simulink model "compare"  (R2025b)
settings: Solver=ode23t  StartTime=0.0  StopTime=4  RelTol=1e-2  AbsTol=1e-2  EnableMultiTasking=on
values from neighbouring files (symbols this model uses):
  k = 2    [compare_init.m]
  N = numel(knee_data)    [display_imu_measurements.m]
  time = 0.08    [compare_init.m]
  X = zeros(N,1)    [display_imu_measurements.m]
  Z = zeros(N,1)    [display_imu_measurements.m]
undefined symbols (not defined in the file or in its folder): foot_radius, ground_offset, hip_max_angle, hip_min_angle, Kaction, knee_max_angle, knee_min_angle, Kpitch, Kroll, Kt, Kv1, Kv2, Ky, Kz, lower_leg, max_a, max_friction_force, max_hip_speed, max_knee_speed, max_magnitude_force, max_torque, max_v, point1, point2, point3, point4, robot_offset, T, Tf, torso, upper_leg, Y
libraries: nesl_utility x88, sm_lib x66, rllib x1
(part 1 of 4)
settings Model: Creator=filip  LastModifiedBy=filip
settings SolverCC: ZeroCrossAlgorithm=Adaptive  MaxZcPerStep=1.0
settings DataIOCC: LimitDataPoints=on  MaxDataPoints=10000
settings OptimizationCC: ReuseModelBlockBuffer=off  LifeSpan=inf
settings DebuggingCC: AlgebraicLoopMsg=none  UnconnectedInputMsg=warning  UnconnectedOutputMsg=warning  UnconnectedLineMsg=warning  AllowSymbolicDim=off  SubsystemReferenceDiagnosticForUnitTest=warning  SFUnexpectedBacktrackingDiag=warning  SFNoUnconditionalDefaultTransitionDiag=warning  SFExecutionAtInitializationDiag=none  ArithmeticOperatorsInVariantConditions=warning
settings ModelReferenceCC: EnableRefExpFcnMdlSchedulingChecks=on
settings SFSimCC: SimUseLocalCustomCode=off  CustomCodeUndefinedFunction=UseInterfaceOnly
settings RTWCC: RTWUseLocalCustomCode=off  GPUComputeCapability=3.5  DLArmComputeVersion=19.05
settings CodeAppCC: StateflowObjectComments=on
settings GRTTargetCC: TargetLangStandard=C89/C90 (ANSI)
settings ConfigComp: CovMetricSettings=dw  CovSaveCumulativeToWorkspaceVar=on  CovSaveSingleToWorkspaceVar=on  CovExternalEMLEnable=off  CovSFcnEnable=off
settings SimscapeCC: SimscapeLogType=all  SimscapeLogSimulationStatistics=on  SimscapeLogDataHistory=10000.0
settings ExplorerConfigSet: InternalSimMechanicsExplorerSettings=|
  | <ExplorerConfiguration>
  | 
  |   <canonicalview>default</canonicalview>
  | 
  |   <TilePanel>
  |     <TileInfo>
  |       <Tiles Columns="1" Count="1" Height="896" Rows="1" Width="1591">
  |         <Row Weight="1"/>
  |         <Column Weight="1"/>
  |         <Tile Height="1" Width="1" X="0" Y="0"/>
  |       </Tiles>
  |     </TileInfo>
  |     <SceneInfo>
  |       <SceneViewer>
  |         <IsThisViewStd>
  |           <IsStandardView>off</IsStandardView>
  |           <StandardViewName>Front</StandardViewName>
  |         </IsThisViewStd>
  |         <BGColor>
  |           <R>1</R>
  |           <G>1</G>
  |           <B>1</B>
  |           <A>1</A>
  |         </BGColor>
  |         <Camera>
  |           <DoPerspective>off</DoPerspective>
  |           <Position>
  |             <X>2.3240540663599489</X>
  |             <Y>-79.864795009647452</Y>
  |             <Z>11.89876292667747</Z>
  |           </Position>
  |           <Center>
  |             <X>0.21287692287567161</X>
  |             <Y>-0.00025892895920284764</Y>
  |             <Z>-0.038859645903780687</Z>
  |           </Center>
  |           <Up>
  |             <X>-0.0013697347920566083</X>
  |             <Y>0.14779550973246389</Y>
  |             <Z>0.98901699233608753</Z>
  |           </Up>
  |           <XLim>0.21304392253015453</XLim>
  |           <YLim>0.21304392253015453</YLim>
  |           <ViewLimDist>0.01</ViewLimDist>
  |         </Camera>
  |       </SceneViewer>
  |     </SceneInfo>
  |   </TilePanel>
  | 
  |   <MechEditorPanel>
  |     <GfxPanelCameraMap/>
  |     <Cameras/>
  |     <VideoCreator>
  |       <IncludeTiles>All</IncludeTiles>
  |       <IncludeTime>on</IncludeTime>
  |       <IncludeWorldFrame>off</IncludeWorldFrame>
  |       <PlaybackSpeedRatio>1</PlaybackSpeedRatio>
  |       <FrameRate>30</FrameRate>
  |       <FrameSize>auto</FrameSize>
  |       <VideoFormat>UncompressedAVI</VideoFormat>
  |     </VideoCreator>
  |   </MechEditorPanel>
  | 
  |   <PlaybackSettings>
  |     <PlaybackSpeedFactor>1</PlaybackSpeedFactor>
  |   </PlaybackSettings>
  | 
  | </ExplorerConfiguration>

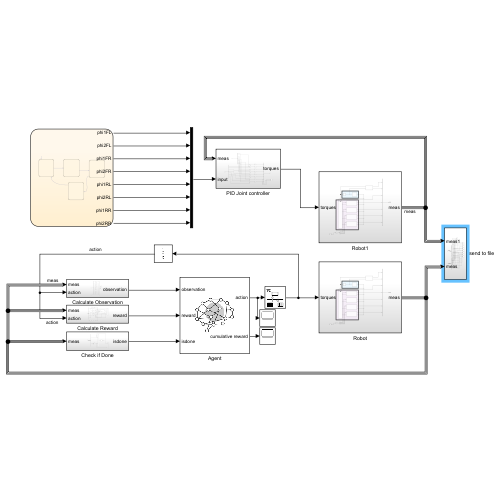
[thumbnail: Simulink's stored preview of the top-level diagram]
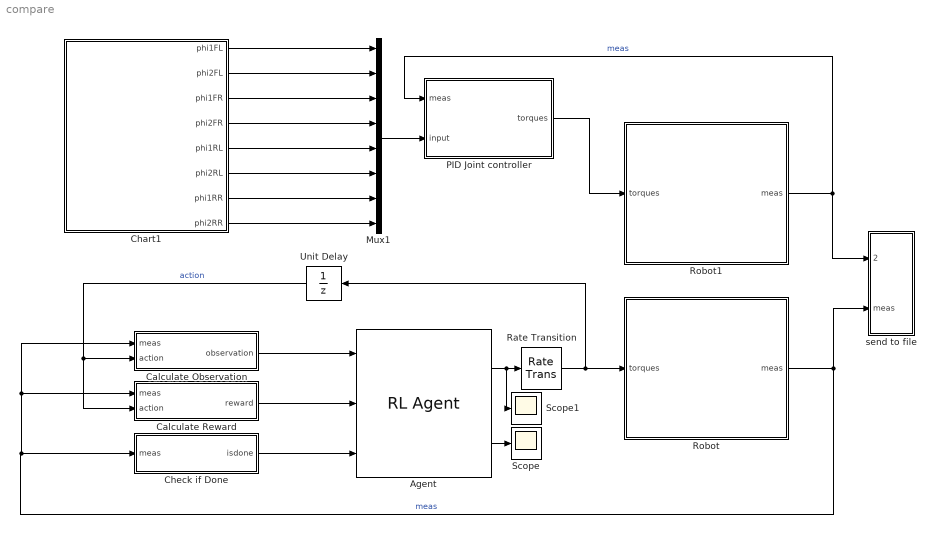
== system compare ==
  Agent : rllib/RL Agent  Agent=agent  ExternalActionAsInput=off  ProvideLastAction=off  ProvideCumRwd=on  TreatAsDirectFeedthrough=on  UseStrictObservationDataTypes=off
  Calculate Observation : Subsystem
  Calculate Reward : Subsystem
  Chart1 : Stateflow chart  TreatAsAtomicUnit=on
  Check if Done : Subsystem
  Mux1 : Mux  Inputs=8
  PID Joint controller : Subsystem
  Rate Transition : RateTransition
  Robot : Subsystem
  Robot1 : Subsystem
  Scope : Scope
      settings: ActiveDisplayYMinimum=-401.67879511543174  ActiveDisplayYMaximum=113.00101014528089
  Scope1 : Scope
      settings: ActiveDisplayYMinimum=-1.0362669645267895  ActiveDisplayYMaximum=0.98271732420125391  DataLoggingVariableName=ScopeData2
  Unit Delay : UnitDelay  SampleTime=-1  HasFrameUpgradeWarning=on
  send to file : Subsystem
      settings: PortSchema="{\"entries\":[{\"content\":{\"sides\":[{\"content\":{},\"type\":\"ConnectorPlacement.EquallySpacedRectSide\",\"uuid\":\"f12f6017-7515-48cd-85fd-4fe04b777209\"},{\"content\":{\"side\":\"RIGHT\"},\"type\":\"ConnectorPlacement.EquallySpacedRectSide\",\"uuid\":\"f5e30d74-7e29-4dc2-8c60-8d5874d82cb8\"},{\"content\":{\"connectorIds\":[\"In1\",\"In2\"],\"side\":\"TOP\"},\"type\":\"ConnectorPlacement.EquallySpacedRectSide\",\"uuid\":\"dbd3eef4-30da-43be-bc56-c6bc5317fe23\"}]},\"type\":\"ConnectorPlacement.EquallySpacedConnector\",\"uuid\":\"0ee742e2-c0d1-4e3d-9783-93de5995511b\"}],\"packageUris\":[\"http://schema.mathworks.com/mf0/Connector/R2020b\"],\"version\":\"1.0\"}"
  wires:
  Calculate Reward/1(reward) -> Agent/2
  Calculate Observation/1(observation) -> Agent/1
  Unit Delay/1 -> Calculate Reward/2(action), Calculate Observation/2(action)  "action"
  Check if Done/1(isdone) -> Agent/3
  Agent/2 -> Scope/1
  Agent/1 -> Rate Transition/1, Scope1/1
  Chart1/6(phi2RL) -> Mux1/6
  Chart1/1(phi1FL) -> Mux1/1
  Chart1/8(phi2RR) -> Mux1/8
  Chart1/3(phi1FR) -> Mux1/3
  Chart1/2(phi2FL) -> Mux1/2
  Chart1/5(phi1RL) -> Mux1/5
  Mux1/1 -> PID Joint controller/2(input)
  Chart1/7(phi1RR) -> Mux1/7
  Chart1/4(phi2FR) -> Mux1/4
  Robot/1(meas) -> Calculate Observation/1(meas), Calculate Reward/1(meas), Check if Done/1(meas), send to file/1(meas)  "meas"
  PID Joint controller/1(torques) -> Robot1/1(torques)
  Rate Transition/1 -> Robot/1(torques), Unit Delay/1
  Robot1/1(meas) -> PID Joint controller/1(meas), send to file/2(meas1)  "meas"

== system compare/Calculate Observation ==
  meas : Inport
  action : Inport  Port=2
  Bus Selector1 : BusSelector  OutputSignals=FL,FR,RL,RR,translation.z,translation.ax,translation.ay,translation.az,rotation.q,translation.vx,translation.vy,translation.vz
  Gain : Gain  Gain=1/(torso(3)/2+upper_leg(1)+lower_leg(1)+2*foot_radius)
  Gain1 : Gain  Gain=1/max_a
  Gain2 : Gain  Gain=1/max_a
  Gain3 : Gain  Gain=1/max_a
  Gain4 : Gain  Gain=1/max_v
  Gain5 : Gain  Gain=1/max_v
  Gain6 : Gain  Gain=1/max_v
  Mux1 : Mux  Inputs=13
  Rate Transition : RateTransition  OutPortSampleTime=T
  Scope : Scope
      settings: ActiveDisplayYMinimum=-2.682935873512565  ActiveDisplayYMaximum=3.0538219458872433  DataLoggingVariableName=ScopeData10
  observe leg : Subsystem
  observe leg1 : Subsystem
  observe leg2 : Subsystem
  observe leg3 : Subsystem
  observation : Outport
  wires:
  meas/1 -> Bus Selector1/1
  Rate Transition/1 -> observation/1
  Mux1/1 -> Scope/1, Rate Transition/1
  Bus Selector1/1 -> observe leg/1(<FL>)  "<FL>"
  Bus Selector1/2 -> observe leg1/1(<FR>)  "<FR>"
  Bus Selector1/3 -> observe leg2/1(<RL>)  "<RL>"
  Bus Selector1/4 -> observe leg3/1(<RR>)  "<RR>"
  observe leg3/1(RR) -> Mux1/4
  observe leg2/1(RL) -> Mux1/3
  observe leg1/1(FR) -> Mux1/2
  Bus Selector1/5 -> Gain/1  "<z>"
  Gain/1 -> Mux1/5
  Bus Selector1/6 -> Gain1/1  "<ax>"
  Bus Selector1/8 -> Gain3/1  "<az>"
  Bus Selector1/7 -> Gain2/1  "<ay>"
  Gain1/1 -> Mux1/6
  Gain2/1 -> Mux1/7
  Gain3/1 -> Mux1/8
  observe leg/1(FL) -> Mux1/1
  Bus Selector1/9 -> Mux1/9  "<q>"
  action/1 -> Mux1/13
  Bus Selector1/10 -> Gain4/1  "<vx>"
  Gain4/1 -> Mux1/10
  Gain5/1 -> Mux1/11
  Bus Selector1/11 -> Gain5/1  "<vy>"
  Bus Selector1/12 -> Gain6/1  "<vz>"
  Gain6/1 -> Mux1/12

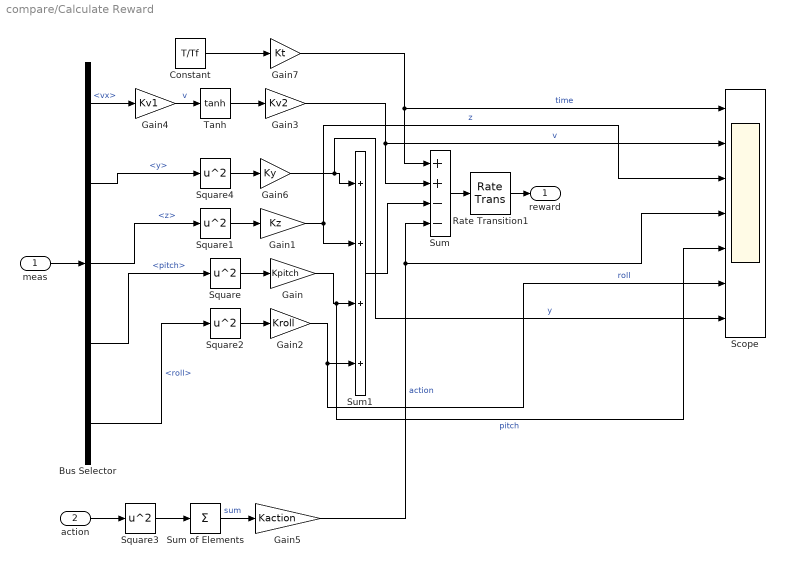
== system compare/Calculate Reward ==
  meas : Inport
  action : Inport  Port=2
  Bus Selector : BusSelector  OutputSignals=translation.vx,translation.y,translation.z,rotation.pitch,rotation.roll
  Constant : Constant  Value=T/Tf
  Gain : Gain  Gain=Kpitch
  Gain1 : Gain  Gain=Kz
  Gain2 : Gain  Gain=Kroll
  Gain3 : Gain  Gain=Kv2
  Gain4 : Gain  Gain=Kv1
  Gain5 : Gain  Gain=Kaction
  Gain6 : Gain  Gain=Ky
  Gain7 : Gain  Gain=Kt
  Rate Transition1 : RateTransition  OutPortSampleTime=T
  Scope : Scope  NumInputPorts=7
      settings: ActiveDisplayYMinimum=-0.47852958861727357  ActiveDisplayYMaximum=1.7073858990610127  DataLoggingVariableName=ScopeData7
  Square{,1..4} (5 alike) : Math  Operator=square
  Sum : Sum  Inputs=++--
  Sum of Elements : Sum  Inputs=+
  Sum1 : Sum  Inputs=++++
  Tanh : Trigonometry  Operator=tanh
  reward : Outport
  wires:
  meas/1 -> Bus Selector/1
  Bus Selector/3 -> Square1/1  "<z>"
  Square1/1 -> Gain1/1
  Bus Selector/2 -> Square4/1  "<y>"
  Square/1 -> Gain/1
  Square2/1 -> Gain2/1
  Gain1/1 -> Scope/3, Sum1/2  "z"
  Gain/1 -> Scope/5, Sum1/3  "pitch"
  Gain2/1 -> Scope/6, Sum1/4  "roll"
  Bus Selector/4 -> Square/1  "<pitch>"
  Bus Selector/5 -> Square2/1  "<roll>"
  Sum1/1 -> Sum/3
  Gain3/1 -> Scope/2, Sum/2  "v"
  Sum/1 -> Rate Transition1/1
  Bus Selector/1 -> Gain4/1  "<vx>"
  Sum of Elements/1 -> Gain5/1  "sum"
  Gain5/1 -> Scope/4, Sum/4  "action"
  Rate Transition1/1 -> reward/1
  action/1 -> Square3/1
  Square3/1 -> Sum of Elements/1
  Tanh/1 -> Gain3/1
  Gain4/1 -> Tanh/1  "v"
  Square4/1 -> Gain6/1
  Gain6/1 -> Scope/7, Sum1/1  "y"
  Constant/1 -> Gain7/1
  Gain7/1 -> Sum/1, Scope/1  "time"

== system compare/Check if Done ==
  meas : Inport
  Bus Selector : BusSelector  OutputSignals=contact,translation.z
  Constant : Constant  Value=ground_offset/3
  Less Than : RelationalOperator  Operator=<  OutDataTypeStr=boolean  RndMeth=Simplest  InputSameDT=off
  OR : Logic  Operator=OR  AllPortsSameDT=off  OutDataTypeStr=boolean
  Rate Transition1 : RateTransition  OutPortSampleTime=T
  Scope : Scope  NumInputPorts=2
      settings: ActiveDisplayYMinimum=-0.073431438758792489  ActiveDisplayYMaximum=1.0063655594055529  DataLoggingVariableName=ScopeData9
  isdone : Outport
  wires:
  meas/1 -> Bus Selector/1
  Bus Selector/1 -> OR/1, Scope/1  "<contact>"
  OR/1 -> Rate Transition1/1
  Rate Transition1/1 -> isdone/1
  Bus Selector/2 -> Less Than/1  "<z>"
  Constant/1 -> Less Than/2
  Less Than/1 -> OR/2, Scope/2  "z"

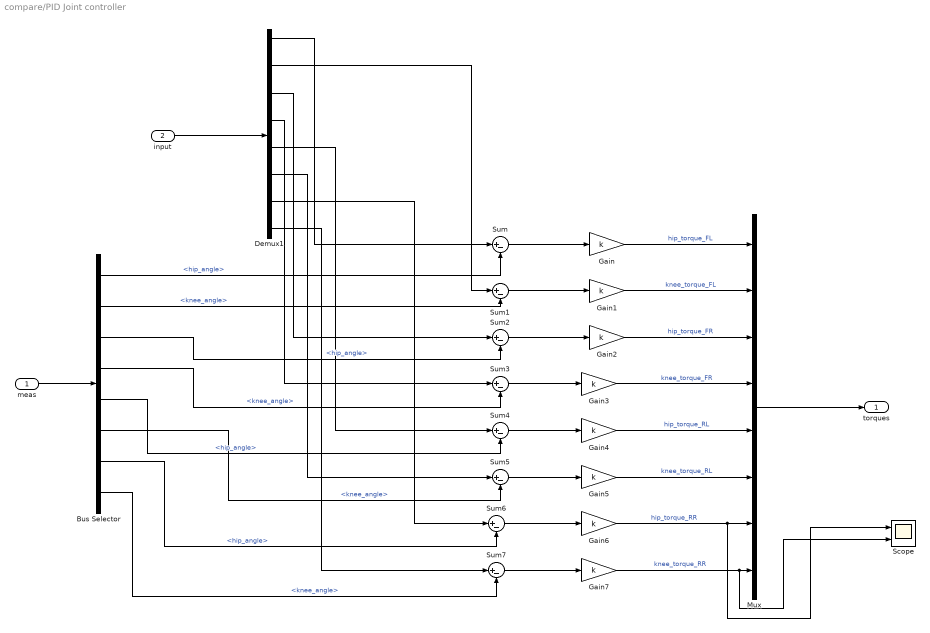
== system compare/PID Joint controller ==
  meas : Inport
  input : Inport  Port=2
  Bus Selector : BusSelector  OutputSignals=FL.hip_angle,FL.knee_angle,FR.hip_angle,FR.knee_angle,RL.hip_angle,RL.knee_angle,RR.hip_angle,RR.knee_angle
  Demux1 : Demux  Outputs=8
  Gain{,1..7} (8 alike) : Gain  Gain=k
  Mux : Mux  Inputs=8
  Scope : Scope  NumInputPorts=2
      settings: ActiveDisplayYMinimum=-0.60150818333502554  ActiveDisplayYMaximum=0.30156485568701297
  Sum{,1..7} (8 alike) : Sum  Inputs=|+-
  torques : Outport
  wires:
  Sum2/1 -> Gain2/1
  Gain4/1 -> Mux/5  "hip_torque_RL"
  Demux1/1 -> Sum/1
  Gain3/1 -> Mux/4  "knee_torque_FR"
  Sum/1 -> Gain/1
  Gain1/1 -> Mux/2  "knee_torque_FL"
  Gain2/1 -> Mux/3  "hip_torque_FR"
  Gain5/1 -> Mux/6  "knee_torque_RL"
  Sum3/1 -> Gain3/1
  Gain/1 -> Mux/1  "hip_torque_FL"
  Demux1/2 -> Sum1/1
  Sum1/1 -> Gain1/1
  Sum7/1 -> Gain7/1
  Demux1/3 -> Sum2/1
  Demux1/4 -> Sum3/1
  Sum4/1 -> Gain4/1
  Sum5/1 -> Gain5/1
  Gain6/1 -> Scope/1, Mux/7  "hip_torque_RR"
  Sum6/1 -> Gain6/1
  Gain7/1 -> Scope/2, Mux/8  "knee_torque_RR"
  Mux/1 -> torques/1
  meas/1 -> Bus Selector/1
  Demux1/5 -> Sum4/1
  Demux1/6 -> Sum5/1
  Demux1/7 -> Sum6/1
  Demux1/8 -> Sum7/1
  input/1 -> Demux1/1
  Bus Selector/1 -> Sum/2  "<hip_angle>"
  Bus Selector/2 -> Sum1/2  "<knee_angle>"
  Bus Selector/3 -> Sum2/2  "<hip_angle>"
  Bus Selector/4 -> Sum3/2  "<knee_angle>"
  Bus Selector/5 -> Sum4/2  "<hip_angle>"
  Bus Selector/6 -> Sum5/2  "<knee_angle>"
  Bus Selector/7 -> Sum6/2  "<hip_angle>"
  Bus Selector/8 -> Sum7/2  "<knee_angle>"

== system compare/Robot ==
  note: Robot Model
  note: Ground
  torques : Inport
  6-DOF Joint : sm_lib/Joints/6-DOF Joint  JointMode=Normal  CompositeWrenchDir=FollowerOnBase  CompositeWrenchFrame=BaseFrame  SenseConstraintForce=off  SenseConstraintTorque=off  SenseTotalForce=off  SenseTotalTorque=off  PxPositionTargetSpecify=off  PxPositionTargetPriority=High  PxPositionTargetValue=0  PxPositionTargetValueUnits=m  PxVelocityTargetSpecify=off  PxVelocityTargetPriority=High  PxVelocityTargetValue=0  PxVelocityTargetValueUnits=m/s  PxEquilibriumPosition=0  PxEquilibriumPositionUnits=m  PxSpringStiffness=0  PxSpringStiffnessUnits=N/m  PxDampingCoefficient=0  PxDampingCoefficientUnits=N/(m/s)  PxLowerLimitSpecify=off  PxLowerLimitBound=-1  PxLowerLimitBoundUnits=m  PxLowerLimitStiffness=1e6  PxLowerLimitStiffnessUnits=N/m  PxLowerLimitDamping=1e3  PxLowerLimitDampingUnits=N/(m/s)  PxLowerLimitTransitionRegionWidth=1e-4  PxLowerLimitTransitionRegionWidthUnits=m  PxUpperLimitSpecify=off  PxUpperLimitBound=1  PxUpperLimitBoundUnits=m  PxUpperLimitStiffness=1e6  PxUpperLimitStiffnessUnits=N/m  PxUpperLimitDamping=1e3  PxUpperLimitDampingUnits=N/(m/s)  PxUpperLimitTransitionRegionWidth=1e-4  PxUpperLimitTransitionRegionWidthUnits=m  PxTorqueActuationMode=NoTorque  PxMotionActuationMode=ComputedMotion  PxSensePosition=off  PxSenseVelocity=off  PxSenseAcceleration=off  PxSenseTorqueForce=off  PxSenseLowerLimitTorqueForce=off  PxSenseUpperLimitTorqueForce=off  PyPositionTargetSpecify=off  PyPositionTargetPriority=High  PyPositionTargetValue=0  PyPositionTargetValueUnits=m  PyVelocityTargetSpecify=off  PyVelocityTargetPriority=High  PyVelocityTargetValue=0  PyVelocityTargetValueUnits=m/s  PyEquilibriumPosition=0  PyEquilibriumPositionUnits=m  PySpringStiffness=0  PySpringStiffnessUnits=N/m  PyDampingCoefficient=0  PyDampingCoefficientUnits=N/(m/s)  PyLowerLimitSpecify=off  PyLowerLimitBound=-1  PyLowerLimitBoundUnits=m  PyLowerLimitStiffness=1e6  PyLowerLimitStiffnessUnits=N/m  PyLowerLimitDamping=1e3  PyLowerLimitDampingUnits=N/(m/s)  PyLowerLimitTransitionRegionWidth=1e-4  PyLowerLimitTransitionRegionWidthUnits=m  PyUpperLimitSpecify=off  PyUpperLimitBound=1  PyUpperLimitBoundUnits=m  PyUpperLimitStiffness=1e6  PyUpperLimitStiffnessUnits=N/m  PyUpperLimitDamping=1e3  PyUpperLimitDampingUnits=N/(m/s)  PyUpperLimitTransitionRegionWidth=1e-4  PyUpperLimitTransitionRegionWidthUnits=m  PyTorqueActuationMode=NoTorque  PyMotionActuationMode=ComputedMotion  PySensePosition=off  PySenseVelocity=off  PySenseAcceleration=off  PySenseTorqueForce=off  PySenseLowerLimitTorqueForce=off  PySenseUpperLimitTorqueForce=off  PzPositionTargetSpecify=off  PzPositionTargetPriority=High  PzPositionTargetValue=0  PzPositionTargetValueUnits=m  PzVelocityTargetSpecify=off  PzVelocityTargetPriority=High  PzVelocityTargetValue=0  PzVelocityTargetValueUnits=m/s  PzEquilibriumPosition=0  PzEquilibriumPositionUnits=m  PzSpringStiffness=0  PzSpringStiffnessUnits=N/m  PzDampingCoefficient=0  PzDampingCoefficientUnits=N/(m/s)  PzLowerLimitSpecify=off  PzLowerLimitBound=-1  PzLowerLimitBoundUnits=m  PzLowerLimitStiffness=1e6  PzLowerLimitStiffnessUnits=N/m  PzLowerLimitDamping=1e3  PzLowerLimitDampingUnits=N/(m/s)  PzLowerLimitTransitionRegionWidth=1e-4  PzLowerLimitTransitionRegionWidthUnits=m  PzUpperLimitSpecify=off  PzUpperLimitBound=1  PzUpperLimitBoundUnits=m  PzUpperLimitStiffness=1e6  PzUpperLimitStiffnessUnits=N/m  PzUpperLimitDamping=1e3  PzUpperLimitDampingUnits=N/(m/s)  PzUpperLimitTransitionRegionWidth=1e-4  PzUpperLimitTransitionRegionWidthUnits=m  PzTorqueActuationMode=NoTorque  PzMotionActuationMode=ComputedMotion  PzSensePosition=off  PzSenseVelocity=off  PzSenseAcceleration=off  PzSenseTorqueForce=off  PzSenseLowerLimitTorqueForce=off  PzSenseUpperLimitTorqueForce=off  SphPositionTargetSpecify=off  SphPositionTargetPriority=High  SphPositionTargetRotationMethod=None  SphPositionTargetFollAlignAxisA=+X  SphPositionTargetBaseAlignAxisA=+Y  SphPositionTargetFollAlignAxisB=+Y  SphPositionTargetBaseAlignAxisB=+Z  SphPositionTargetRotationStandardAxis=+Z  SphPositionTargetRotationAngle=0  SphPositionTargetRotationAngleUnits=deg  SphPositionTargetRotationArbitraryAxis=[0 0 1]  SphPositionTargetRotationSequenceAxes=FollowerAxes  SphPositionTargetRotationSequence=XYX  SphPositionTargetRotationSequenceAngles=[0 0 0]  SphPositionTargetRotationSequenceAnglesUnits=deg  SphPositionTargetRotationMatrix=[1 0 0;0 1 0;0 0 1]  SphPositionTargetQuaternion=[1 0 0 0]  SphVelocityTargetSpecify=off  SphVelocityTargetPriority=High  SphVelocityTargetValue=[0 0 0]  SphVelocityTargetValueUnits=deg/s  SphVelocityTargetInFollowerFrame=on  SphEqPosRotationMethod=None  SphEqPosFollAlignAxisA=+X  SphEqPosBaseAlignAxisA=+Y  SphEqPosFollAlignAxisB=+Y  SphEqPosBaseAlignAxisB=+Z  SphEqPosRotationStandardAxis=+Z  SphEqPosRotationAngle=0  SphEqPosRotationAngleUnits=deg  SphEqPosRotationArbitraryAxis=[0 0 1]  SphEqPosRotationSequenceAxes=FollowerAxes  SphEqPosRotationSequence=XYX  SphEqPosRotationSequenceAngles=[0 0 0]  SphEqPosRotationSequenceAnglesUnits=deg  SphEqPosRotationMatrix=[1 0 0;0 1 0;0 0 1]  SphEqPosQuaternion=[1 0 0 0]  SphSpringStiffness=0  SphSpringStiffnessUnits=N*m/deg  SphDampingCoefficient=0  SphDampingCoefficientUnits=N*m/(deg/s)  SphLowerLimitSpecify=off  SphLowerLimitBound=15  SphLowerLimitBoundUnits=deg  SphLowerLimitStiffness=1e4  SphLowerLimitStiffnessUnits=N*m/deg  SphLowerLimitDamping=10  SphLowerLimitDampingUnits=N*m/(deg/s)  SphLowerLimitTransitionRegionWidth=0.1  SphLowerLimitTransitionRegionWidthUnits=deg  SphUpperLimitSpecify=off  SphUpperLimitBound=45  SphUpperLimitBoundUnits=deg  SphUpperLimitStiffness=1e4  SphUpperLimitStiffnessUnits=N*m/deg  SphUpperLimitDamping=10  SphUpperLimitDampingUnits=N*m/(deg/s)  SphUpperLimitTransitionRegionWidth=0.1  SphUpperLimitTransitionRegionWidthUnits=deg  SphTorqueActuationMode=NoTorque  SphActuateTorqueX=off  SphActuateTorqueY=off  SphActuateTorqueZ=off  SphActuateTorque=off  SphActuationFrame=BaseFrame  SphSensePosition=off  SphSenseVelocityX=off  SphSenseVelocityY=off  SphSenseVelocityZ=off  SphSenseVelocity=off  SphSenseAccelerationX=off  SphSenseAccelerationY=off  SphSenseAccelerationZ=off  SphSenseAcceleration=off  SphSenseLowerLimitTorqueMag=off  SphSenseUpperLimitTorqueMag=off  SphSensingFrame=BaseFrame
  Body Measurment : Subsystem
  Bus Creator : BusCreator  Inputs=7
  Demux : Demux
  Front Left Leg : Subsystem
      settings: PortSchema="{\"entries\":[{\"content\":{\"sides\":[{\"content\":{\"connectorIds\":[\"LConn1\",\"In1\"]},\"type\":\"ConnectorPlacement.EquallySpacedRectSide\",\"uuid\":\"67cc346d-8093-4a90-beea-ad102c28a529\"},{\"content\":{\"connectorIds\":[\"RConn1\",\"Out1\"],\"side\":\"RIGHT\"},\"type\":\"ConnectorPlacement.EquallySpacedRectSide\",\"uuid\":\"a41fbdac-a3bc-454a-9a02-c1548b06e168\"},{\"content\":{\"side\":\"TOP\"},\"type\":\"ConnectorPlacement.EquallySpacedRectSide\",\"uuid\":\"2db3de25-17b9-42a2-b258-04f424c8657a\"}]},\"type\":\"ConnectorPlacement.EquallySpacedConnector\",\"uuid\":\"8d839d8f-2b1b-4b58-b696-304cf56daaed\"}],\"packageUris\":[\"http://schema.mathworks.com/mf0/Connector/R2020b\"],\"version\":\"1.0\"}"
  Front Right Leg : Subsystem
      settings: PortSchema="{\"entries\":[{\"content\":{\"sides\":[{\"content\":{\"connectorIds\":[\"LConn1\",\"In1\"]},\"type\":\"ConnectorPlacement.EquallySpacedRectSide\",\"uuid\":\"34c80378-d001-4ef7-8c50-56da40a680d3\"},{\"content\":{\"connectorIds\":[\"RConn1\",\"Out1\"],\"side\":\"RIGHT\"},\"type\":\"ConnectorPlacement.EquallySpacedRectSide\",\"uuid\":\"d8c47c46-5f9d-4ebc-b52e-d8bb210754e6\"},{\"content\":{\"side\":\"TOP\"},\"type\":\"ConnectorPlacement.EquallySpacedRectSide\",\"uuid\":\"9923bc19-0faa-4da1-9dcb-df221e5d47f7\"}]},\"type\":\"ConnectorPlacement.EquallySpacedConnector\",\"uuid\":\"13843bdb-d0bb-4acc-95de-2d753d5922a7\"}],\"packageUris\":[\"http://schema.mathworks.com/mf0/Connector/R2020b\"],\"version\":\"1.0\"}"
  Gain : Gain  Gain=max_torque
  Rear Left Leg : Subsystem
      settings: PortSchema="{\"entries\":[{\"content\":{\"sides\":[{\"content\":{\"connectorIds\":[\"LConn1\",\"In1\"]},\"type\":\"ConnectorPlacement.EquallySpacedRectSide\",\"uuid\":\"34c80378-d001-4ef7-8c50-56da40a680d3\"},{\"content\":{\"connectorIds\":[\"RConn1\",\"Out1\"],\"side\":\"RIGHT\"},\"type\":\"ConnectorPlacement.EquallySpacedRectSide\",\"uuid\":\"d8c47c46-5f9d-4ebc-b52e-d8bb210754e6\"},{\"content\":{\"side\":\"TOP\"},\"type\":\"ConnectorPlacement.EquallySpacedRectSide\",\"uuid\":\"9923bc19-0faa-4da1-9dcb-df221e5d47f7\"}]},\"type\":\"ConnectorPlacement.EquallySpacedConnector\",\"uuid\":\"13843bdb-d0bb-4acc-95de-2d753d5922a7\"}],\"packageUris\":[\"http://schema.mathworks.com/mf0/Connector/R2020b\"],\"version\":\"1.0\"}"
  Rear Right Leg : Subsystem
      settings: PortSchema="{\"entries\":[{\"content\":{\"sides\":[{\"content\":{\"connectorIds\":[\"LConn1\",\"In1\"]},\"type\":\"ConnectorPlacement.EquallySpacedRectSide\",\"uuid\":\"34c80378-d001-4ef7-8c50-56da40a680d3\"},{\"content\":{\"connectorIds\":[\"RConn1\",\"Out1\"],\"side\":\"RIGHT\"},\"type\":\"ConnectorPlacement.EquallySpacedRectSide\",\"uuid\":\"d8c47c46-5f9d-4ebc-b52e-d8bb210754e6\"},{\"content\":{\"side\":\"TOP\"},\"type\":\"ConnectorPlacement.EquallySpacedRectSide\",\"uuid\":\"9923bc19-0faa-4da1-9dcb-df221e5d47f7\"}]},\"type\":\"ConnectorPlacement.EquallySpacedConnector\",\"uuid\":\"13843bdb-d0bb-4acc-95de-2d753d5922a7\"}],\"packageUris\":[\"http://schema.mathworks.com/mf0/Connector/R2020b\"],\"version\":\"1.0\"}"
  Torso : Subsystem
      settings: PortSchema="{\"entries\":[{\"content\":{\"sides\":[{\"content\":{\"connectorIds\":[\"LConn1\",\"LConn2\",\"LConn3\",\"LConn4\"]},\"type\":\"ConnectorPlacement.EquallySpacedRectSide\",\"uuid\":\"8c53a05f-c94a-44be-b209-a034cec6561e\"},{\"content\":{\"side\":\"RIGHT\"},\"type\":\"ConnectorPlacement.EquallySpacedRectSide\",\"uuid\":\"a3c22973-bf74-4661-9744-7bfaa32719ac\"},{\"content\":{\"connectorIds\":[\"Out1\",\"LConn5\",\"LConn6\"],\"side\":\"TOP\"},\"type\":\"ConnectorPlacement.EquallySpacedRectSide\",\"uuid\":\"da2dd510-6694-4077-b588-65723e1f355d\"}]},\"type\":\"ConnectorPlacement.EquallySpacedConnector\",\"uuid\":\"e4e4bf1c-8f02-4a77-9d3b-bb8def7996fd\"}],\"packageUris\":[\"http://schema.mathworks.com/mf0/Connector/R2020b\"],\"version\":\"1.0\"}"
  World and Ground : Subsystem
  meas : Outport
  wires:
  Demux/2 -> Front Right Leg/1(torques)
  Demux/3 -> Rear Left Leg/1(torques)
  Demux/4 -> Rear Right Leg/1(torques)
  Demux/1 -> Front Left Leg/1(torques)
  Front Left Leg/1(FL) -> Bus Creator/4  "FL"
  Bus Creator/1 -> meas/1
  Front Right Leg/1(FR) -> Bus Creator/5  "FR"
  Rear Left Leg/1(RL) -> Bus Creator/6  "RL"
  Rear Right Leg/1(RR) -> Bus Creator/7  "RR"
  Torso/1(contact) -> Bus Creator/3  "contact"
  Body Measurment/2(rotation) -> Bus Creator/2  "rotation"
  Body Measurment/1(translation) -> Bus Creator/1  "translation"
  Gain/1 -> Demux/1
  torques/1 -> Gain/1
  connections:
  Front Left Leg/RConn1 -- World and Ground/LConn1 -- Torso/LConn6 -- Front Right Leg/RConn1 -- Rear Right Leg/RConn1 -- Rear Left Leg/RConn1
  Rear Right Leg/LConn1 -- Torso/LConn4
  Body Measurment/LConn2 -- 6-DOF Joint/LConn1 -- World and Ground/RConn1
  Front Right Leg/LConn1 -- Torso/LConn2
  6-DOF Joint/RConn1 -- Body Measurment/LConn1 -- Torso/LConn5
  Torso/LConn1 -- Front Left Leg/LConn1
  Rear Left Leg/LConn1 -- Torso/LConn3

== system compare/Robot1 ==
  note: Robot Model
  note: Ground
  torques : Inport
  6-DOF Joint : sm_lib/Joints/6-DOF Joint  JointMode=Normal  CompositeWrenchDir=FollowerOnBase  CompositeWrenchFrame=BaseFrame  SenseConstraintForce=off  SenseConstraintTorque=off  SenseTotalForce=off  SenseTotalTorque=off  PxPositionTargetSpecify=off  PxPositionTargetPriority=High  PxPositionTargetValue=0  PxPositionTargetValueUnits=m  PxVelocityTargetSpecify=off  PxVelocityTargetPriority=High  PxVelocityTargetValue=0  PxVelocityTargetValueUnits=m/s  PxEquilibriumPosition=0  PxEquilibriumPositionUnits=m  PxSpringStiffness=0  PxSpringStiffnessUnits=N/m  PxDampingCoefficient=0  PxDampingCoefficientUnits=N/(m/s)  PxLowerLimitSpecify=off  PxLowerLimitBound=-1  PxLowerLimitBoundUnits=m  PxLowerLimitStiffness=1e6  PxLowerLimitStiffnessUnits=N/m  PxLowerLimitDamping=1e3  PxLowerLimitDampingUnits=N/(m/s)  PxLowerLimitTransitionRegionWidth=1e-4  PxLowerLimitTransitionRegionWidthUnits=m  PxUpperLimitSpecify=off  PxUpperLimitBound=1  PxUpperLimitBoundUnits=m  PxUpperLimitStiffness=1e6  PxUpperLimitStiffnessUnits=N/m  PxUpperLimitDamping=1e3  PxUpperLimitDampingUnits=N/(m/s)  PxUpperLimitTransitionRegionWidth=1e-4  PxUpperLimitTransitionRegionWidthUnits=m  PxTorqueActuationMode=NoTorque  PxMotionActuationMode=ComputedMotion  PxSensePosition=off  PxSenseVelocity=off  PxSenseAcceleration=off  PxSenseTorqueForce=off  PxSenseLowerLimitTorqueForce=off  PxSenseUpperLimitTorqueForce=off  PyPositionTargetSpecify=off  PyPositionTargetPriority=High  PyPositionTargetValue=0  PyPositionTargetValueUnits=m  PyVelocityTargetSpecify=off  PyVelocityTargetPriority=High  PyVelocityTargetValue=0  PyVelocityTargetValueUnits=m/s  PyEquilibriumPosition=0  PyEquilibriumPositionUnits=m  PySpringStiffness=0  PySpringStiffnessUnits=N/m  PyDampingCoefficient=0  PyDampingCoefficientUnits=N/(m/s)  PyLowerLimitSpecify=off  PyLowerLimitBound=-1  PyLowerLimitBoundUnits=m  PyLowerLimitStiffness=1e6  PyLowerLimitStiffnessUnits=N/m  PyLowerLimitDamping=1e3  PyLowerLimitDampingUnits=N/(m/s)  PyLowerLimitTransitionRegionWidth=1e-4  PyLowerLimitTransitionRegionWidthUnits=m  PyUpperLimitSpecify=off  PyUpperLimitBound=1  PyUpperLimitBoundUnits=m  PyUpperLimitStiffness=1e6  PyUpperLimitStiffnessUnits=N/m  PyUpperLimitDamping=1e3  PyUpperLimitDampingUnits=N/(m/s)  PyUpperLimitTransitionRegionWidth=1e-4  PyUpperLimitTransitionRegionWidthUnits=m  PyTorqueActuationMode=NoTorque  PyMotionActuationMode=ComputedMotion  PySensePosition=off  PySenseVelocity=off  PySenseAcceleration=off  PySenseTorqueForce=off  PySenseLowerLimitTorqueForce=off  PySenseUpperLimitTorqueForce=off  PzPositionTargetSpecify=off  PzPositionTargetPriority=High  PzPositionTargetValue=0  PzPositionTargetValueUnits=m  PzVelocityTargetSpecify=off  PzVelocityTargetPriority=High  PzVelocityTargetValue=0  PzVelocityTargetValueUnits=m/s  PzEquilibriumPosition=0  PzEquilibriumPositionUnits=m  PzSpringStiffness=0  PzSpringStiffnessUnits=N/m  PzDampingCoefficient=0  PzDampingCoefficientUnits=N/(m/s)  PzLowerLimitSpecify=off  PzLowerLimitBound=-1  PzLowerLimitBoundUnits=m  PzLowerLimitStiffness=1e6  PzLowerLimitStiffnessUnits=N/m  PzLowerLimitDamping=1e3  PzLowerLimitDampingUnits=N/(m/s)  PzLowerLimitTransitionRegionWidth=1e-4  PzLowerLimitTransitionRegionWidthUnits=m  PzUpperLimitSpecify=off  PzUpperLimitBound=1  PzUpperLimitBoundUnits=m  PzUpperLimitStiffness=1e6  PzUpperLimitStiffnessUnits=N/m  PzUpperLimitDamping=1e3  PzUpperLimitDampingUnits=N/(m/s)  PzUpperLimitTransitionRegionWidth=1e-4  PzUpperLimitTransitionRegionWidthUnits=m  PzTorqueActuationMode=NoTorque  PzMotionActuationMode=ComputedMotion  PzSensePosition=off  PzSenseVelocity=off  PzSenseAcceleration=off  PzSenseTorqueForce=off  PzSenseLowerLimitTorqueForce=off  PzSenseUpperLimitTorqueForce=off  SphPositionTargetSpecify=off  SphPositionTargetPriority=High  SphPositionTargetRotationMethod=None  SphPositionTargetFollAlignAxisA=+X  SphPositionTargetBaseAlignAxisA=+Y  SphPositionTargetFollAlignAxisB=+Y  SphPositionTargetBaseAlignAxisB=+Z  SphPositionTargetRotationStandardAxis=+Z  SphPositionTargetRotationAngle=0  SphPositionTargetRotationAngleUnits=deg  SphPositionTargetRotationArbitraryAxis=[0 0 1]  SphPositionTargetRotationSequenceAxes=FollowerAxes  SphPositionTargetRotationSequence=XYX  SphPositionTargetRotationSequenceAngles=[0 0 0]  SphPositionTargetRotationSequenceAnglesUnits=deg  SphPositionTargetRotationMatrix=[1 0 0;0 1 0;0 0 1]  SphPositionTargetQuaternion=[1 0 0 0]  SphVelocityTargetSpecify=off  SphVelocityTargetPriority=High  SphVelocityTargetValue=[0 0 0]  SphVelocityTargetValueUnits=deg/s  SphVelocityTargetInFollowerFrame=on  SphEqPosRotationMethod=None  SphEqPosFollAlignAxisA=+X  SphEqPosBaseAlignAxisA=+Y  SphEqPosFollAlignAxisB=+Y  SphEqPosBaseAlignAxisB=+Z  SphEqPosRotationStandardAxis=+Z  SphEqPosRotationAngle=0  SphEqPosRotationAngleUnits=deg  SphEqPosRotationArbitraryAxis=[0 0 1]  SphEqPosRotationSequenceAxes=FollowerAxes  SphEqPosRotationSequence=XYX  SphEqPosRotationSequenceAngles=[0 0 0]  SphEqPosRotationSequenceAnglesUnits=deg  SphEqPosRotationMatrix=[1 0 0;0 1 0;0 0 1]  SphEqPosQuaternion=[1 0 0 0]  SphSpringStiffness=0  SphSpringStiffnessUnits=N*m/deg  SphDampingCoefficient=0  SphDampingCoefficientUnits=N*m/(deg/s)  SphLowerLimitSpecify=off  SphLowerLimitBound=15  SphLowerLimitBoundUnits=deg  SphLowerLimitStiffness=1e4  SphLowerLimitStiffnessUnits=N*m/deg  SphLowerLimitDamping=10  SphLowerLimitDampingUnits=N*m/(deg/s)  SphLowerLimitTransitionRegionWidth=0.1  SphLowerLimitTransitionRegionWidthUnits=deg  SphUpperLimitSpecify=off  SphUpperLimitBound=45  SphUpperLimitBoundUnits=deg  SphUpperLimitStiffness=1e4  SphUpperLimitStiffnessUnits=N*m/deg  SphUpperLimitDamping=10  SphUpperLimitDampingUnits=N*m/(deg/s)  SphUpperLimitTransitionRegionWidth=0.1  SphUpperLimitTransitionRegionWidthUnits=deg  SphTorqueActuationMode=NoTorque  SphActuateTorqueX=off  SphActuateTorqueY=off  SphActuateTorqueZ=off  SphActuateTorque=off  SphActuationFrame=BaseFrame  SphSensePosition=off  SphSenseVelocityX=off  SphSenseVelocityY=off  SphSenseVelocityZ=off  SphSenseVelocity=off  SphSenseAccelerationX=off  SphSenseAccelerationY=off  SphSenseAccelerationZ=off  SphSenseAcceleration=off  SphSenseLowerLimitTorqueMag=off  SphSenseUpperLimitTorqueMag=off  SphSensingFrame=BaseFrame
  Body Measurment : Subsystem
  Bus Creator : BusCreator  Inputs=7
  Demux : Demux
  Front Left Leg : Subsystem
      settings: PortSchema="{\"entries\":[{\"content\":{\"sides\":[{\"content\":{\"connectorIds\":[\"LConn1\",\"In1\"]},\"type\":\"ConnectorPlacement.EquallySpacedRectSide\",\"uuid\":\"67cc346d-8093-4a90-beea-ad102c28a529\"},{\"content\":{\"connectorIds\":[\"RConn1\",\"Out1\"],\"side\":\"RIGHT\"},\"type\":\"ConnectorPlacement.EquallySpacedRectSide\",\"uuid\":\"a41fbdac-a3bc-454a-9a02-c1548b06e168\"},{\"content\":{\"side\":\"TOP\"},\"type\":\"ConnectorPlacement.EquallySpacedRectSide\",\"uuid\":\"2db3de25-17b9-42a2-b258-04f424c8657a\"}]},\"type\":\"ConnectorPlacement.EquallySpacedConnector\",\"uuid\":\"8d839d8f-2b1b-4b58-b696-304cf56daaed\"}],\"packageUris\":[\"http://schema.mathworks.com/mf0/Connector/R2020b\"],\"version\":\"1.0\"}"
  Front Right Leg : Subsystem
      settings: PortSchema="{\"entries\":[{\"content\":{\"sides\":[{\"content\":{\"connectorIds\":[\"LConn1\",\"In1\"]},\"type\":\"ConnectorPlacement.EquallySpacedRectSide\",\"uuid\":\"34c80378-d001-4ef7-8c50-56da40a680d3\"},{\"content\":{\"connectorIds\":[\"RConn1\",\"Out1\"],\"side\":\"RIGHT\"},\"type\":\"ConnectorPlacement.EquallySpacedRectSide\",\"uuid\":\"d8c47c46-5f9d-4ebc-b52e-d8bb210754e6\"},{\"content\":{\"side\":\"TOP\"},\"type\":\"ConnectorPlacement.EquallySpacedRectSide\",\"uuid\":\"9923bc19-0faa-4da1-9dcb-df221e5d47f7\"}]},\"type\":\"ConnectorPlacement.EquallySpacedConnector\",\"uuid\":\"13843bdb-d0bb-4acc-95de-2d753d5922a7\"}],\"packageUris\":[\"http://schema.mathworks.com/mf0/Connector/R2020b\"],\"version\":\"1.0\"}"
  Gain : Gain  Gain=max_torque
  Rear Left Leg : Subsystem
      settings: PortSchema="{\"entries\":[{\"content\":{\"sides\":[{\"content\":{\"connectorIds\":[\"LConn1\",\"In1\"]},\"type\":\"ConnectorPlacement.EquallySpacedRectSide\",\"uuid\":\"34c80378-d001-4ef7-8c50-56da40a680d3\"},{\"content\":{\"connectorIds\":[\"RConn1\",\"Out1\"],\"side\":\"RIGHT\"},\"type\":\"ConnectorPlacement.EquallySpacedRectSide\",\"uuid\":\"d8c47c46-5f9d-4ebc-b52e-d8bb210754e6\"},{\"content\":{\"side\":\"TOP\"},\"type\":\"ConnectorPlacement.EquallySpacedRectSide\",\"uuid\":\"9923bc19-0faa-4da1-9dcb-df221e5d47f7\"}]},\"type\":\"ConnectorPlacement.EquallySpacedConnector\",\"uuid\":\"13843bdb-d0bb-4acc-95de-2d753d5922a7\"}],\"packageUris\":[\"http://schema.mathworks.com/mf0/Connector/R2020b\"],\"version\":\"1.0\"}"
  Rear Right Leg : Subsystem
      settings: PortSchema="{\"entries\":[{\"content\":{\"sides\":[{\"content\":{\"connectorIds\":[\"LConn1\",\"In1\"]},\"type\":\"ConnectorPlacement.EquallySpacedRectSide\",\"uuid\":\"34c80378-d001-4ef7-8c50-56da40a680d3\"},{\"content\":{\"connectorIds\":[\"RConn1\",\"Out1\"],\"side\":\"RIGHT\"},\"type\":\"ConnectorPlacement.EquallySpacedRectSide\",\"uuid\":\"d8c47c46-5f9d-4ebc-b52e-d8bb210754e6\"},{\"content\":{\"side\":\"TOP\"},\"type\":\"ConnectorPlacement.EquallySpacedRectSide\",\"uuid\":\"9923bc19-0faa-4da1-9dcb-df221e5d47f7\"}]},\"type\":\"ConnectorPlacement.EquallySpacedConnector\",\"uuid\":\"13843bdb-d0bb-4acc-95de-2d753d5922a7\"}],\"packageUris\":[\"http://schema.mathworks.com/mf0/Connector/R2020b\"],\"version\":\"1.0\"}"
  Torso : Subsystem
      settings: PortSchema="{\"entries\":[{\"content\":{\"sides\":[{\"content\":{\"connectorIds\":[\"LConn1\",\"LConn2\",\"LConn3\",\"LConn4\"]},\"type\":\"ConnectorPlacement.EquallySpacedRectSide\",\"uuid\":\"8c53a05f-c94a-44be-b209-a034cec6561e\"},{\"content\":{\"side\":\"RIGHT\"},\"type\":\"ConnectorPlacement.EquallySpacedRectSide\",\"uuid\":\"a3c22973-bf74-4661-9744-7bfaa32719ac\"},{\"content\":{\"connectorIds\":[\"Out1\",\"LConn5\",\"LConn6\"],\"side\":\"TOP\"},\"type\":\"ConnectorPlacement.EquallySpacedRectSide\",\"uuid\":\"da2dd510-6694-4077-b588-65723e1f355d\"}]},\"type\":\"ConnectorPlacement.EquallySpacedConnector\",\"uuid\":\"e4e4bf1c-8f02-4a77-9d3b-bb8def7996fd\"}],\"packageUris\":[\"http://schema.mathworks.com/mf0/Connector/R2020b\"],\"version\":\"1.0\"}"
  World and Ground : Subsystem
  meas : Outport
  wires:
  Demux/2 -> Front Right Leg/1(torques)
  Demux/3 -> Rear Left Leg/1(torques)
  Demux/4 -> Rear Right Leg/1(torques)
  Demux/1 -> Front Left Leg/1(torques)
  Front Left Leg/1(FL) -> Bus Creator/4  "FL"
  Bus Creator/1 -> meas/1
  Front Right Leg/1(FR) -> Bus Creator/5  "FR"
  Rear Left Leg/1(RL) -> Bus Creator/6  "RL"
  Rear Right Leg/1(RR) -> Bus Creator/7  "RR"
  Torso/1(contact) -> Bus Creator/3  "contact"
  Body Measurment/2(rotation) -> Bus Creator/2  "rotation"
  Body Measurment/1(translation) -> Bus Creator/1  "translation"
  Gain/1 -> Demux/1
  torques/1 -> Gain/1
  connections:
  Front Left Leg/RConn1 -- World and Ground/LConn1 -- Torso/LConn6 -- Front Right Leg/RConn1 -- Rear Right Leg/RConn1 -- Rear Left Leg/RConn1
  Rear Right Leg/LConn1 -- Torso/LConn4
  Body Measurment/LConn2 -- 6-DOF Joint/LConn1 -- World and Ground/RConn1
  Front Right Leg/LConn1 -- Torso/LConn2
  6-DOF Joint/RConn1 -- Body Measurment/LConn1 -- Torso/LConn5
  Torso/LConn1 -- Front Left Leg/LConn1
  Rear Left Leg/LConn1 -- Torso/LConn3

== system compare/send to file ==
  meas : Inport
  meas1 : Inport  Port=2
  Bus Selector : BusSelector  OutputSignals=translation.x,translation.z,translation.vx,FL.knee_angle,FL.hip_angle,FR.knee_angle,FR.hip_angle,RL.knee_angle,RL.hip_angle,RR.knee_angle,RR.hip_angle,translation.ax,rotation.pitch,rotation.roll,rotation.yaw
  Bus Selector1 : BusSelector  OutputSignals=translation.x,translation.z,translation.vx,FL.knee_angle,FL.hip_angle,FR.knee_angle,FR.hip_angle,RL.knee_angle,RL.hip_angle,RR.knee_angle,RR.hip_angle,translation.ax,rotation.pitch,rotation.roll,rotation.yaw
  Scope{,1..14} (15 alike) : Scope  NumInputPorts=2
      Scope settings: ActiveDisplayYMinimum=-2.1231695967448174  ActiveDisplayYMaximum=6.1996949033692985  DataLoggingVariableName=x_
      Scope1 settings: ActiveDisplayYMinimum=-0.060989059903898586  ActiveDisplayYMaximum=0.067425736242765155  DataLoggingVariableName=z_
      Scope10 settings: DataLoggingVariableName=hip_angle_dataFL
      Scope11 settings: DataLoggingVariableName=knee_angle_dataFR
      Scope12 settings: DataLoggingVariableName=hip_angle_dataFR
      Scope13 settings: DataLoggingVariableName=knee_angle_dataRL
      Scope14 settings: DataLoggingVariableName=hip_angle_dataRL
      Scope2 settings: ActiveDisplayYMinimum=-2.6304119067580847  ActiveDisplayYMaximum=5.2842672335749379  DataLoggingVariableName=v_
      Scope3 settings: ActiveDisplayYMinimum=1.3903180165239624  ActiveDisplayYMaximum=2.3143968931245986  DataLoggingVariableName=knee_angle_dataRR
      Scope4 settings: ActiveDisplayYMinimum=-1.4796641533615718  ActiveDisplayYMaximum=0.239354913188759  DataLoggingVariableName=hip_angle_dataRR
      Scope5 settings: DataLoggingVariableName=a_
      Scope6 settings: DataLoggingVariableName=pitch_
      Scope7 settings: DataLoggingVariableName=roll_
      Scope8 settings: DataLoggingVariableName=yaw_
      Scope9 settings: ActiveDisplayYMinimum=1.5090205096222653  ActiveDisplayYMaximum=2.1219933370843109  DataLoggingVariableName=knee_angle_dataFL
  wires:
  meas/1 -> Bus Selector/1
  Bus Selector/1 -> Scope/1  "<x>"
  Bus Selector/2 -> Scope1/1  "<z>"
  Bus Selector/3 -> Scope2/1  "<vx>"
  Bus Selector1/3 -> Scope2/2  "<vx>"
  Bus Selector1/2 -> Scope1/2  "<z>"
  Bus Selector1/1 -> Scope/2  "<x>"
  meas1/1 -> Bus Selector1/1
  Bus Selector/10 -> Scope3/1  "<knee_angle>"
  Bus Selector/11 -> Scope4/1  "<hip_angle>"
  Bus Selector1/10 -> Scope3/2  "<knee_angle>"
  Bus Selector1/11 -> Scope4/2  "<hip_angle>"
  Bus Selector/12 -> Scope5/1  "<ax>"
  Bus Selector1/12 -> Scope5/2  "<ax>"
  Bus Selector/13 -> Scope6/1  "<pitch>"
  Bus Selector1/13 -> Scope6/2  "<pitch>"
  Bus Selector/14 -> Scope7/1  "<roll>"
  Bus Selector1/14 -> Scope7/2  "<roll>"
  Bus Selector/15 -> Scope8/1  "<yaw>"
  Bus Selector1/15 -> Scope8/2  "<yaw>"
  Bus Selector/4 -> Scope9/1  "<knee_angle>"
  Bus Selector1/4 -> Scope9/2  "<knee_angle>"
  Bus Selector/5 -> Scope10/1  "<hip_angle>"
  Bus Selector1/5 -> Scope10/2  "<hip_angle>"
  Bus Selector/6 -> Scope11/1  "<knee_angle>"
  Bus Selector1/6 -> Scope11/2  "<knee_angle>"
  Bus Selector/7 -> Scope12/1  "<hip_angle>"
  Bus Selector1/7 -> Scope12/2  "<hip_angle>"
  Bus Selector/8 -> Scope13/1  "<knee_angle>"
  Bus Selector1/8 -> Scope13/2  "<knee_angle>"
  Bus Selector/9 -> Scope14/1  "<hip_angle>"
  Bus Selector1/9 -> Scope14/2  "<hip_angle>"

== system compare/Calculate Observation/observe leg ==
  <FL> : Inport
  Bias : Bias  Bias=-hip_min_angle  SaturateOnIntegerOverflow=off
  Bias1 : Bias  Bias=-knee_min_angle  SaturateOnIntegerOverflow=off
  Bus Selector2 : BusSelector  OutputSignals=hip_speed,hip_angle,knee_speed,knee_angle,force_magnitude,friction_force_magnitude
  Gain : Gain  Gain=1/max_hip_speed
  Gain1 : Gain  Gain=1/(hip_max_angle - hip_min_angle)
  Gain2 : Gain  Gain=1/max_knee_speed
  Gain3 : Gain  Gain=1/(knee_max_angle - knee_min_angle)
  Gain4 : Gain  Gain=1/max_magnitude_force
  Gain5 : Gain  Gain=1/max_friction_force
  Mux1 : Mux  Inputs=6
  FL : Outport
  wires:
  Gain/1 -> Mux1/1
  Gain1/1 -> Mux1/2
  Bus Selector2/6 -> Gain5/1  "<friction_force_magnitude>"
  Bus Selector2/4 -> Bias1/1  "<knee_angle>"
  Bus Selector2/5 -> Gain4/1  "<force_magnitude>"
  Gain2/1 -> Mux1/3
  Gain3/1 -> Mux1/4
  Gain4/1 -> Mux1/5
  Bus Selector2/2 -> Bias/1  "<hip_angle>"
  Mux1/1 -> FL/1  "FL"
  Bias/1 -> Gain1/1
  Bus Selector2/3 -> Gain2/1  "<knee_speed>"
  Gain5/1 -> Mux1/6
  Bias1/1 -> Gain3/1
  <FL>/1 -> Bus Selector2/1
  Bus Selector2/1 -> Gain/1  "<hip_speed>"

== system compare/Calculate Observation/observe leg1 ==
  <FR> : Inport
  Bias : Bias  Bias=-hip_min_angle  SaturateOnIntegerOverflow=off
  Bias1 : Bias  Bias=-knee_min_angle  SaturateOnIntegerOverflow=off
  Bus Selector2 : BusSelector  OutputSignals=hip_speed,hip_angle,knee_speed,knee_angle,force_magnitude,friction_force_magnitude
  Gain : Gain  Gain=1/max_hip_speed
  Gain1 : Gain  Gain=1/(hip_max_angle - hip_min_angle)
  Gain2 : Gain  Gain=1/max_knee_speed
  Gain3 : Gain  Gain=1/(knee_max_angle - knee_min_angle)
  Gain4 : Gain  Gain=1/max_magnitude_force
  Gain5 : Gain  Gain=1/max_friction_force
  Mux1 : Mux  Inputs=6
  FR : Outport
  wires:
  Gain/1 -> Mux1/1
  Gain1/1 -> Mux1/2
  Bus Selector2/6 -> Gain5/1  "<friction_force_magnitude>"
  Bus Selector2/4 -> Bias1/1  "<knee_angle>"
  Bus Selector2/5 -> Gain4/1  "<force_magnitude>"
  Gain2/1 -> Mux1/3
  Gain3/1 -> Mux1/4
  Gain4/1 -> Mux1/5
  Bus Selector2/2 -> Bias/1  "<hip_angle>"
  Mux1/1 -> FR/1  "FR"
  Bias/1 -> Gain1/1
  Bus Selector2/3 -> Gain2/1  "<knee_speed>"
  Gain5/1 -> Mux1/6
  Bias1/1 -> Gain3/1
  <FR>/1 -> Bus Selector2/1
  Bus Selector2/1 -> Gain/1  "<hip_speed>"

== system compare/Calculate Observation/observe leg2 ==
  <RL> : Inport
  Bias : Bias  Bias=-hip_min_angle  SaturateOnIntegerOverflow=off
  Bias1 : Bias  Bias=-knee_min_angle  SaturateOnIntegerOverflow=off
  Bus Selector2 : BusSelector  OutputSignals=hip_speed,hip_angle,knee_speed,knee_angle,force_magnitude,friction_force_magnitude
  Gain : Gain  Gain=1/max_hip_speed
  Gain1 : Gain  Gain=1/(hip_max_angle - hip_min_angle)
  Gain2 : Gain  Gain=1/max_knee_speed
  Gain3 : Gain  Gain=1/(knee_max_angle - knee_min_angle)
  Gain4 : Gain  Gain=1/max_magnitude_force
  Gain5 : Gain  Gain=1/max_friction_force
  Mux1 : Mux  Inputs=6
  RL : Outport
  wires:
  Gain/1 -> Mux1/1
  Gain1/1 -> Mux1/2
  Bus Selector2/6 -> Gain5/1  "<friction_force_magnitude>"
  Bus Selector2/4 -> Bias1/1  "<knee_angle>"
  Bus Selector2/5 -> Gain4/1  "<force_magnitude>"
  Gain2/1 -> Mux1/3
  Gain3/1 -> Mux1/4
  Gain4/1 -> Mux1/5
  Bus Selector2/2 -> Bias/1  "<hip_angle>"
  Mux1/1 -> RL/1  "RL"
  Bias/1 -> Gain1/1
  Bus Selector2/3 -> Gain2/1  "<knee_speed>"
  Gain5/1 -> Mux1/6
  Bias1/1 -> Gain3/1
  <RL>/1 -> Bus Selector2/1
  Bus Selector2/1 -> Gain/1  "<hip_speed>"

== system compare/Calculate Observation/observe leg3 ==
  <RR> : Inport
  Bias : Bias  Bias=-hip_min_angle  SaturateOnIntegerOverflow=off
  Bias1 : Bias  Bias=-knee_min_angle  SaturateOnIntegerOverflow=off
  Bus Selector2 : BusSelector  OutputSignals=hip_speed,hip_angle,knee_speed,knee_angle,force_magnitude,friction_force_magnitude
  Gain : Gain  Gain=1/max_hip_speed
  Gain1 : Gain  Gain=1/(hip_max_angle - hip_min_angle)
  Gain2 : Gain  Gain=1/max_knee_speed
  Gain3 : Gain  Gain=1/(knee_max_angle - knee_min_angle)
  Gain4 : Gain  Gain=1/max_magnitude_force
  Gain5 : Gain  Gain=1/max_friction_force
  Mux1 : Mux  Inputs=6
  RR : Outport
  wires:
  Gain/1 -> Mux1/1
  Gain1/1 -> Mux1/2
  Bus Selector2/6 -> Gain5/1  "<friction_force_magnitude>"
  Bus Selector2/4 -> Bias1/1  "<knee_angle>"
  Bus Selector2/5 -> Gain4/1  "<force_magnitude>"
  Gain2/1 -> Mux1/3
  Gain3/1 -> Mux1/4
  Gain4/1 -> Mux1/5
  Bus Selector2/2 -> Bias/1  "<hip_angle>"
  Mux1/1 -> RR/1  "RR"
  Bias/1 -> Gain1/1
  Bus Selector2/3 -> Gain2/1  "<knee_speed>"
  Gain5/1 -> Mux1/6
  Bias1/1 -> Gain3/1
  <RR>/1 -> Bus Selector2/1
  Bus Selector2/1 -> Gain/1  "<hip_speed>"

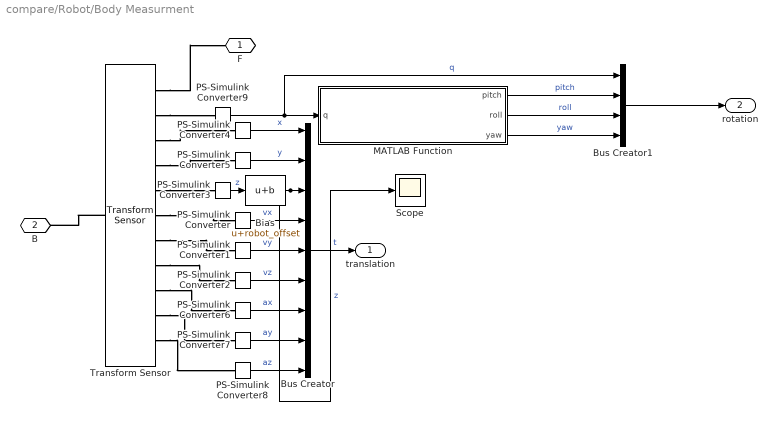
== system compare/Robot/Body Measurment ==
  Bias : Bias  Bias=robot_offset  SaturateOnIntegerOverflow=off
  Bus Creator : BusCreator  Inputs=9
  Bus Creator1 : BusCreator  Inputs=4
  MATLAB Function : MATLAB Function  TreatAsAtomicUnit=on
  PS-Simulink Converter{,1..9} (10 alike) : nesl_utility/PS-Simulink Converter  PhysicalDomain=network_engine_domain  SubClassName=ps_output  LeftPortType=input  RightPortType=output  PseudoPeriodic=off  Frequencies=[]  VectorFormat=inherit  Unit=inherit  AffineConversion=off
  Scope : Scope
      settings: ActiveDisplayYMinimum=-1  ActiveDisplayYMaximum=1  DataLoggingVariableName=ScopeData8
  Transform Sensor : sm_lib/Frames and Transforms/Transform Sensor  MeasurementFrame=World  RotationSequence=XYX  SenseAngle=off  SenseAxis=off  SenseQ=on  SenseR=off  SenseRotationSequence=off  SenseOmegaX=off  SenseOmegaY=off  SenseOmegaZ=off  SenseOmega=off  SenseQDot=off  SenseRDot=off  SenseRotationSequenceDot=off  SenseAlphaX=off  SenseAlphaY=off  SenseAlphaZ=off  SenseAlpha=off  SenseQDDot=off  SenseRDDot=off  SenseX=on  SenseY=on  SenseZ=on  SenseXYZ=off  SenseRad=off  SenseAzim=off  SenseDist=off  SenseInc=off  SenseXDot=on  SenseYDot=on  SenseZDot=on  SenseXYZDot=off  SenseRadDot=off  SenseAzimDot=off  SenseDistDot=off  SenseIncDot=off  SenseXDDot=on  SenseYDDot=on  SenseZDDot=on  SenseXYZDDot=off  SenseRadDDot=off  SenseAzimDDot=off  SenseDistDDot=off  SenseIncDDot=off
  F : PMIOPort  Side=Left
  B : PMIOPort  Port=2  Side=Left
  translation : Outport
  rotation : Outport  Port=2
  wires:
  PS-Simulink Converter4/1 -> Bus Creator/1  "x"
  PS-Simulink Converter/1 -> Bus Creator/4  "vx"
  PS-Simulink Converter5/1 -> Bus Creator/2  "y"
  PS-Simulink Converter2/1 -> Bus Creator/6  "vz"
  PS-Simulink Converter1/1 -> Bus Creator/5  "vy"
  Bus Creator/1 -> translation/1  "t"
  PS-Simulink Converter7/1 -> Bus Creator/8  "ay"
  PS-Simulink Converter8/1 -> Bus Creator/9  "az"
  PS-Simulink Converter6/1 -> Bus Creator/7  "ax"
  PS-Simulink Converter9/1 -> Bus Creator1/1, MATLAB Function/1(q)  "q"
  Bus Creator1/1 -> rotation/1
  MATLAB Function/1(pitch) -> Bus Creator1/2  "pitch"
  MATLAB Function/2(roll) -> Bus Creator1/3  "roll"
  MATLAB Function/3(yaw) -> Bus Creator1/4  "yaw"
  PS-Simulink Converter3/1 -> Bias/1  "z"
  Bias/1 -> Scope/1, Bus Creator/3  "z"
  connections:
  Transform Sensor/RConn6 -- PS-Simulink Converter/LConn1
  Transform Sensor/RConn7 -- PS-Simulink Converter1/LConn1
  Transform Sensor/RConn8 -- PS-Simulink Converter2/LConn1
  Transform Sensor/RConn1 -- F/RConn1
  Transform Sensor/RConn3 -- PS-Simulink Converter4/LConn1
  Transform Sensor/RConn5 -- PS-Simulink Converter3/LConn1
  Transform Sensor/RConn4 -- PS-Simulink Converter5/LConn1
  Transform Sensor/LConn1 -- B/RConn1
  Transform Sensor/RConn11 -- PS-Simulink Converter8/LConn1
  Transform Sensor/RConn9 -- PS-Simulink Converter6/LConn1
  Transform Sensor/RConn10 -- PS-Simulink Converter7/LConn1
  Transform Sensor/RConn2 -- PS-Simulink Converter9/LConn1
